simulink model "FaultOfFeeder"  (R2019a)
settings: Solver=ode1  StartTime=0.0  StopTime=2.5  FixedStep=Ts_Power  RelTol=1e-3
PostLoadFcn:
  | %% Init for wind PnO models - global system parameters
  | OVERRIDE_SSN_MEMORY_LIMIT=1;
  | Ts=50e-6;
  | % Ts=50e-10;
  | Ts_Power=Ts;
  | Ts_Control=2*Ts;
  | freq = 50;
  | Fnom=freq;
  | Vac=400e3;
InitFcn:
  | %% Init for wind PnO models - global system parameters
  | OVERRIDE_SSN_MEMORY_LIMIT=1;
  | Ts=50e-6;
  | % Ts=50e-10;
  | Ts_Power=Ts;
  | Ts_Control=2*Ts;
  | freq = 50;
  | Fnom=freq;
  | Vac=225e3;
values from neighbouring files (symbols this model uses):
  ohl_posCap = (0.01e-006)*12    (= 1.2e-07)    [variable.m]
  ohl_posInd = (1.15e-3)/12    (= 9.58333333333e-05)    [variable.m]
  ohl_posR = 0.069/12    (= 0.00575)    [variable.m]
  ohl_zeroCap = (0.004e-006)*12    (= 4.8e-08)    [variable.m]
  ohl_zeroInd = (2.86e-3)/12    (= 0.000238333333333)    [variable.m]
  ohl_zeroR = 0.1725/12    (= 0.014375)    [variable.m]
  sub_posCap = sub_posCap*6    (= 9.6e-07)    [variable.m]
  sub_posInd = sub_posInd/6    (= 0.000233333333333)    [variable.m]
  sub_posR = sub_posR/6    (= 0.006)    [variable.m]
  sub_zeroCap = sub_zeroCap*6    (= 3.84e-07)    [variable.m]
  sub_zeroInd = sub_zeroInd/6    (= 0.000583333333333)    [variable.m]
  sub_zeroR = sub_zeroR/6    (= 0.015)    [variable.m]
  transfo_L1 = 0.05999374    [variable.m]
  transfo_L2 = 0.05999374    [variable.m]
  transfo_R1 = 0.000866667    [variable.m]
  transfo_R2 = 0.00086667    [variable.m]
undefined symbols (not defined in the file or in its folder): D1, D11, Delta, den, DiscIntNeverNeededParam, dx, find_system, gcbh, num, out_Buses, out_WindFarms, sps_rtmsupport
libraries: powerlib x202, simulink x96, powerlib_meascontrol x96, elements x52, eeSinusoidalMeasurement x51, simulink_extras x42, spsVIMeasurementModel x36, eePowerMeasurement x16
(part 13 of 24)

== system FaultOfFeeder/SM_WT1/Transformer differential element 1/Differential Relay/logic block ==
  IDa1 : Inport
  IRa1 : Inport  Port=2
  IDa2 : Inport  Port=3
  IDa5 : Inport  Port=4
  Bias Characteristic - A3 : elements/Bias Characteristic  BC=[ 0 0; x1 y1; x2 y2 ]  fs=freq*32
  Data Type Conversion : DataTypeConversion  OutDataTypeStr=boolean
  Gain : Gain  Gain=c2  SaturateOnIntegerOverflow=on  OutDataTypeStr=Inherit: Same as input  ParamDataTypeStr=Inherit: Same as input
  Gain1 : Gain  Gain=c5  SaturateOnIntegerOverflow=on  OutDataTypeStr=Inherit: Same as input  ParamDataTypeStr=Inherit: Same as input
  Logical Operator : Logic  Inputs=4
  Logical Operator1 : Logic  Operator=OR
  compare{,1..3} (4 alike) : RelationalOperator  Operator=>  RndMeth=Nearest  InputSameDT=on
  pickup : Constant  Value=pickup
  unbiased : Constant  Value=unbiased
  Trip A : Outport  VectorParamsAs1DForOutWhenUnconnected=on
  wires:
  Gain/1 -> compare/1
  Gain1/1 -> compare1/1
  pickup/1 -> compare2/2
  unbiased/1 -> compare3/2
  IDa2/1 -> compare/2
  IDa5/1 -> compare1/2
  Logical Operator1/1 -> Trip A/1
  Logical Operator/1 -> Logical Operator1/1
  compare3/1 -> Logical Operator1/2
  compare/1 -> Logical Operator/2
  compare1/1 -> Logical Operator/3
  compare2/1 -> Logical Operator/4
  IRa1/1 -> Bias Characteristic - A3/2
  IDa1/1 -> Bias Characteristic - A3/1, Gain/1, Gain1/1, compare2/1, compare3/1
  Bias Characteristic - A3/1 -> Data Type Conversion/1
  Data Type Conversion/1 -> Logical Operator/1

== system FaultOfFeeder/SM_WT1/Transformer differential element 1/Differential Relay/logic block1 ==
  IDb1 : Inport
  IRb1 : Inport  Port=2
  IDb2 : Inport  Port=3
  IDb5 : Inport  Port=4
  Bias Characteristic - A3 : elements/Bias Characteristic  BC=[ 0 0; x1 y1; x2 y2 ]  fs=freq*32
  Data Type Conversion : DataTypeConversion  OutDataTypeStr=boolean
  Gain : Gain  Gain=c2  SaturateOnIntegerOverflow=on  OutDataTypeStr=Inherit: Same as input  ParamDataTypeStr=Inherit: Same as input
  Gain1 : Gain  Gain=c5  SaturateOnIntegerOverflow=on  OutDataTypeStr=Inherit: Same as input  ParamDataTypeStr=Inherit: Same as input
  Logical Operator : Logic  Inputs=4
  Logical Operator1 : Logic  Operator=OR
  compare{,1..3} (4 alike) : RelationalOperator  Operator=>  RndMeth=Nearest  InputSameDT=on
  pickup : Constant  Value=pickup
  unbiased : Constant  Value=unbiased
  Trip B : Outport  VectorParamsAs1DForOutWhenUnconnected=on
  wires:
  IDb1/1 -> compare3/1, compare2/1, Gain1/1, Gain/1, Bias Characteristic - A3/1
  IRb1/1 -> Bias Characteristic - A3/2
  compare2/1 -> Logical Operator/4
  compare1/1 -> Logical Operator/3
  compare/1 -> Logical Operator/2
  compare3/1 -> Logical Operator1/2
  Logical Operator/1 -> Logical Operator1/1
  Logical Operator1/1 -> Trip B/1
  IDb5/1 -> compare1/2
  IDb2/1 -> compare/2
  unbiased/1 -> compare3/2
  pickup/1 -> compare2/2
  Gain1/1 -> compare1/1
  Gain/1 -> compare/1
  Bias Characteristic - A3/1 -> Data Type Conversion/1
  Data Type Conversion/1 -> Logical Operator/1

== system FaultOfFeeder/SM_WT1/Transformer differential element 1/Differential Relay/logic block2 ==
  IDc1 : Inport
  IRc1 : Inport  Port=2
  IDc2 : Inport  Port=3
  IDc5 : Inport  Port=4
  Bias Characteristic - A3 : elements/Bias Characteristic  BC=[ 0 0; x1 y1; x2 y2 ]  fs=freq*32
  Data Type Conversion : DataTypeConversion  OutDataTypeStr=boolean
  Gain : Gain  Gain=c2  SaturateOnIntegerOverflow=on  OutDataTypeStr=Inherit: Same as input  ParamDataTypeStr=Inherit: Same as input
  Gain1 : Gain  Gain=c5  SaturateOnIntegerOverflow=on  OutDataTypeStr=Inherit: Same as input  ParamDataTypeStr=Inherit: Same as input
  Logical Operator : Logic  Inputs=4
  Logical Operator1 : Logic  Operator=OR
  compare{,1..3} (4 alike) : RelationalOperator  Operator=>  RndMeth=Nearest  InputSameDT=on
  pickup : Constant  Value=pickup
  unbiased : Constant  Value=unbiased
  Trip C : Outport  VectorParamsAs1DForOutWhenUnconnected=on
  wires:
  Gain/1 -> compare/1
  Gain1/1 -> compare1/1
  pickup/1 -> compare2/2
  unbiased/1 -> compare3/2
  IDc2/1 -> compare/2
  IDc5/1 -> compare1/2
  Logical Operator1/1 -> Trip C/1
  Logical Operator/1 -> Logical Operator1/1
  compare3/1 -> Logical Operator1/2
  compare/1 -> Logical Operator/2
  compare1/1 -> Logical Operator/3
  compare2/1 -> Logical Operator/4
  IRc1/1 -> Bias Characteristic - A3/2
  IDc1/1 -> Bias Characteristic - A3/1, Gain/1, Gain1/1, compare2/1, compare3/1
  Bias Characteristic - A3/1 -> Data Type Conversion/1
  Data Type Conversion/1 -> Logical Operator/1

== system FaultOfFeeder/SM_WT1/Transformer differential element 1/Signal Processing1/Differential and restraining currents ==
  IHA : Inport
  IHB : Inport  Port=2
  IHC : Inport  Port=3
  IXA : Inport  Port=4
  IXB : Inport  Port=5
  IXC : Inport  Port=6
   {,1..5} (6 alike) : elements/   fo=freq  window_size=32  harmonic=[1 2 3 4 5]
  -VG-2- : elements/-VG-2-  trtype=wye - delta  vector=1  Vh=vp  Vx=vs  nCTH=cth  nCTX=ctx
  DAB{8..12} (5 alike) : elements/DAB  filter=off  approx=Bessel  order=2  numerator=[]  denominator=[]  freq=360  resdis=off  vertres=12  xmax=10  winsize=32  G=1.0  fs=freq*32
  DAB7 : elements/DAB  filter=on  approx=Bessel  order=2  numerator=[]  denominator=[]  freq=360  resdis=off  vertres=12  xmax=10  winsize=32  G=1.0  fs=freq*32
  Terminator_{6..7,9..10,12..13,15..26} (18 alike) : Terminator
  iDa1 : Outport  VectorParamsAs1DForOutWhenUnconnected=on
  iDa2 : Outport  Port=2  VectorParamsAs1DForOutWhenUnconnected=on
  iDa5 : Outport  Port=3  VectorParamsAs1DForOutWhenUnconnected=on
  iDb1 : Outport  Port=4  VectorParamsAs1DForOutWhenUnconnected=on
  iDb2 : Outport  Port=5  VectorParamsAs1DForOutWhenUnconnected=on
  iDb5 : Outport  Port=6  VectorParamsAs1DForOutWhenUnconnected=on
  iDc1 : Outport  Port=7  VectorParamsAs1DForOutWhenUnconnected=on
  iDc2 : Outport  Port=8  VectorParamsAs1DForOutWhenUnconnected=on
  iDc5 : Outport  Port=9  VectorParamsAs1DForOutWhenUnconnected=on
  iRa1 : Outport  Port=10  VectorParamsAs1DForOutWhenUnconnected=on
  iRb1 : Outport  Port=11  VectorParamsAs1DForOutWhenUnconnected=on
  iRc1 : Outport  Port=12  VectorParamsAs1DForOutWhenUnconnected=on
  wires:
  -VG-2-/1 -> DAB7/1
  -VG-2-/2 -> DAB8/1
  -VG-2-/3 -> DAB9/1
  -VG-2-/4 -> DAB10/1
  -VG-2-/5 -> DAB11/1
  -VG-2-/6 -> DAB12/1
  " 2"/3 -> Terminator_12/1
  " 2"/4 -> Terminator_13/1
  " 4"/5 -> Terminator_21/1
  DAB9/1 -> " 2"/1
  " 5"/2 -> Terminator_26/1
  " 5"/3 -> Terminator_23/1
  " 5"/4 -> Terminator_24/1
  " 5"/5 -> Terminator_25/1
  DAB12/1 -> " 5"/1
  " 4"/3 -> Terminator_19/1
  " 4"/2 -> Terminator_22/1
  DAB11/1 -> " 4"/1
  " 4"/4 -> Terminator_20/1
  " 3"/3 -> Terminator_15/1
  " 3"/4 -> Terminator_16/1
  " 3"/5 -> Terminator_17/1
  " 3"/2 -> Terminator_18/1
  DAB10/1 -> " 3"/1
  " 2"/1 -> iDc1/1
  " 2"/2 -> iDc2/1
  " 2"/5 -> iDc5/1
  " 3"/1 -> iRa1/1
  " 4"/1 -> iRb1/1
  " 5"/1 -> iRc1/1
  IXC/1 -> -VG-2-/6
  IXB/1 -> -VG-2-/5
  IXA/1 -> -VG-2-/4
  IHC/1 -> -VG-2-/3
  IHB/1 -> -VG-2-/2
  IHA/1 -> -VG-2-/1
  " "/4 -> Terminator_6/1
  " "/3 -> Terminator_7/1
  DAB7/1 -> " "/1
  " "/1 -> iDa1/1
  " "/2 -> iDa2/1
  " "/5 -> iDa5/1
  " 1"/3 -> Terminator_9/1
  " 1"/4 -> Terminator_10/1
  " 1"/1 -> iDb1/1
  " 1"/2 -> iDb2/1
  " 1"/5 -> iDb5/1
  DAB8/1 -> " 1"/1

== system FaultOfFeeder/SM_WT1/Transformer differential element 1/Signal Processing1/Phasor-magnitude (IR) ==
  IRa1 : Inport
  IRb1 : Inport  Port=2
  IRC1 : Inport  Port=3
  Demux : Demux  Outputs=2
  Demux1 : Demux  Outputs=2
  Demux2 : Demux  Outputs=2
  Terminator_10 : Terminator
  Terminator_8 : Terminator
  Terminator_9 : Terminator
  1 freq. : Outport  VectorParamsAs1DForOutWhenUnconnected=on
  1 freq.1 : Outport  Port=2  VectorParamsAs1DForOutWhenUnconnected=on
  1 freq.2 : Outport  Port=3  VectorParamsAs1DForOutWhenUnconnected=on
  wires:
  Demux/2 -> Terminator_8/1
  Demux/1 -> 1 freq./1
  IRa1/1 -> Demux/1
  Demux1/2 -> Terminator_9/1
  Demux1/1 -> 1 freq.1/1
  IRb1/1 -> Demux1/1
  Demux2/2 -> Terminator_10/1
  Demux2/1 -> 1 freq.2/1
  IRC1/1 -> Demux2/1

== system FaultOfFeeder/SM_WT1/Transformer differential element 1/Signal Processing1/phasor-magnitude (IDa) ==
  In1 : Inport
  In2 : Inport  Port=2
  In3 : Inport  Port=3
  Demux : Demux  Outputs=2
  Demux1 : Demux  Outputs=2
  Demux2 : Demux  Outputs=2
  Terminator_11 : Terminator
  Terminator_14 : Terminator
  Terminator_8 : Terminator
  1 freq. : Outport  VectorParamsAs1DForOutWhenUnconnected=on
  2 freq. : Outport  Port=2  VectorParamsAs1DForOutWhenUnconnected=on
  5 freq. : Outport  Port=3  VectorParamsAs1DForOutWhenUnconnected=on
  wires:
  In2/1 -> Demux1/1
  In3/1 -> Demux2/1
  In1/1 -> Demux/1
  Demux1/2 -> Terminator_11/1
  Demux2/2 -> Terminator_14/1
  Demux1/1 -> 2 freq./1
  Demux2/1 -> 5 freq./1
  Demux/2 -> Terminator_8/1
  Demux/1 -> 1 freq./1

== system FaultOfFeeder/SM_WT1/Transformer differential element 1/Signal Processing1/phasor-magnitude (iDb) ==
  In1 : Inport
  In2 : Inport  Port=2
  In3 : Inport  Port=3
  Demux : Demux  Outputs=2
  Demux1 : Demux  Outputs=2
  Demux2 : Demux  Outputs=2
  Terminator_11 : Terminator
  Terminator_14 : Terminator
  Terminator_8 : Terminator
  1 freq. : Outport  VectorParamsAs1DForOutWhenUnconnected=on
  2 freq. : Outport  Port=2  VectorParamsAs1DForOutWhenUnconnected=on
  5 freq. : Outport  Port=3  VectorParamsAs1DForOutWhenUnconnected=on
  wires:
  Demux1/2 -> Terminator_11/1
  Demux2/2 -> Terminator_14/1
  Demux/2 -> Terminator_8/1
  Demux/1 -> 1 freq./1
  In1/1 -> Demux/1
  Demux1/1 -> 2 freq./1
  In2/1 -> Demux1/1
  Demux2/1 -> 5 freq./1
  In3/1 -> Demux2/1

== system FaultOfFeeder/SM_WT1/Transformer differential element 1/Signal Processing1/phasor-magnitude (iDc) ==
  In1 : Inport
  In2 : Inport  Port=2
  In3 : Inport  Port=3
  Demux : Demux  Outputs=2
  Demux1 : Demux  Outputs=2
  Demux2 : Demux  Outputs=2
  Terminator_11 : Terminator
  Terminator_14 : Terminator
  Terminator_8 : Terminator
  1 freq. : Outport  VectorParamsAs1DForOutWhenUnconnected=on
  2 freq. : Outport  Port=2  VectorParamsAs1DForOutWhenUnconnected=on
  5 freq. : Outport  Port=3  VectorParamsAs1DForOutWhenUnconnected=on
  wires:
  In3/1 -> Demux2/1
  Demux2/1 -> 5 freq./1
  In2/1 -> Demux1/1
  Demux1/1 -> 2 freq./1
  In1/1 -> Demux/1
  Demux/1 -> 1 freq./1
  Demux/2 -> Terminator_8/1
  Demux2/2 -> Terminator_14/1
  Demux1/2 -> Terminator_11/1

== system FaultOfFeeder/SM_WT1/Wind Type IV Detailed v2.1 - 1/AC fault ride though characteristic/Triggered Subsystem ==
  In1 : Inport
  Trigger : TriggerPort  VariantControl=Variant
  Time_trigger_FRT : Outport  VectorParamsAs1DForOutWhenUnconnected=on
  wires:
  In1/1 -> Time_trigger_FRT/1

== system FaultOfFeeder/SM_WT1/Wind Type IV Detailed v2.1 - 1/Control/2 sample av. ==
  in : Inport
  Delay : Delay  DelayLength=1  InitialCondition=Init_value  SampleTime=Ts
  Delay1 : Delay  DelayLength=1  InitialCondition=Init_value  SampleTime=Ts
  Gain : Gain  Gain=0.5
  Sum1 : Sum  Inputs=|++
  out : Outport
  wires:
  Gain/1 -> out/1
  in/1 -> Delay/1
  Delay1/1 -> Sum1/2
  Sum1/1 -> Gain/1
  Delay/1 -> Delay1/1, Sum1/1

== system FaultOfFeeder/SM_WT1/Wind Type IV Detailed v2.1 - 1/Control/Measurement and Transformation ==
  note: Block forever in case of
      | persistent system overvoltage
  note: Check for normal frequency
  note: Protection against unstable grid events
  note: Check for normal voltage
  note: Outputs
  note: PLL
  note: P,Q & V
  note: Inputs / filtering
  Vabc_grid : Inport
  Iabc_gc : Inport  Port=2
  IL : Inport  Port=3
  Vdc : Inport  Port=4
  Qref : Inport  Port=5
  C_var_filter : Gain  Gain=C_var_filter  SaturateOnIntegerOverflow=on  OutDataTypeStr=Inherit: Same as input  ParamDataTypeStr=Inherit: Same as input
  C_var_filter/Q : Gain  Gain=C_var_filter/Q_filter  SaturateOnIntegerOverflow=on  OutDataTypeStr=Inherit: Same as input  ParamDataTypeStr=Inherit: Same as input
  Compare To Constant1 : simulink/Logic and Bit Operations/Compare To Constant  relop=<  const=0.5  OutDataTypeStr=boolean
  Compare To Constant3 : simulink/Logic and Bit Operations/Compare To Constant  relop=<  const=0.5  OutDataTypeStr=boolean
  Constant : Constant  Value=Vnom
  Constant1 : Constant  Value=Vnom/sqrt(3)*sqrt(2)
  Constant2 : Constant  Value=20
  Constant3 : Constant  SampleTime=Ts
  Constant4 : Constant  SampleTime=Ts
  Digital Clock1 : DigitalClock  SampleTime=Ts
  Digital Clock2 : DigitalClock  SampleTime=Ts
  Discrete 3-phase PLL-Driven Positive-Sequence Active & Reactive Power : Subsystem  mask(Discrete 3-phase PLL-Driven Positive-Sequence Active & Reactive Power){Finit=freq, Fmin=freq*45/60, Par_Vinit=[Vnom/sqrt(3)*sqrt(2) 30], Par_Iinit=[Pnom/sqrt(3)/Vnom*sqrt(2) -10], Ts=Ts}
      mask prompts: Finit "Initial frequency (Hz):"; Fmin "Minimum frequency (Hz):"; Par_Vinit "Voltage initial input: [ Mag  Phase(Degrees) ]"; Par_Iinit "Current initial input: [ Mag  Phase(Degrees) ]"; Ts "Sample time:"
      mask help:
      | This discrete block measures the 3-phase active power P and reactive power Q  associated with a periodic set of 3-phase voltages and currents which may contain harmonics. P and Q are calculated by evaluating the fundamental values (positive-sequence) of the input voltages and currents with a running window over one cycle of the specified frequency (port Freq).
      |  Input port "Sin_Cos" (a two-dimension signal) provides the reference frame required for the computation.
      |
      | input 1: must give the frequency of the fundamental (Hz)
      | Input 2: must contain a  [sin(wt)  cos(wt)] two dimension signal , where w is the rotation speed (rad/s) of the reference frame used for the computation..
      | input 3: Vectorized 3-phase  instantaneous voltage (Vabc)
      | input 4: Vectorized 3-phase instantaneous current (Iabc)
      |
      | Output 1: Vector [Mag_V Mag_I] of the fundamental values (Magnitude) of the voltage & current (peak values of the positive-sequence)
      | Output 2: 3-phase PQ measurement vector [P(W) Q (var)] evaluated at the specified frequency. Current flowing into an RL circuit will produce  positive active and reactive powers.
      |
      | For the first cycle of simulation, the outputs are held constant using the values specified by the parameters "Initial input".
      | he value of the parameter "Minimum frequency" is used to determine the buffer size of the "Variable Transport Delay" block found inside this subsystem.
      mask init:
      | power_initmask();
      settings: OpenFcn=power_openblockproxy();
  Divide : Product  Inputs=*/
  Filter : Subsystem  mask{Freq=Freq_filter, Zeta=Zeta_filter, Ts=Ts}
      mask prompts: Freq "Cut-off frequency (Hz):"; Zeta "Damping factor Zeta:"; Ts "Sample time"
  Gain : Gain  Gain=1.4
  Less Than : RelationalOperator  Operator=>  OutDataTypeStr=boolean  RndMeth=Simplest
  Less Than1 : RelationalOperator  Operator=>  OutDataTypeStr=boolean  RndMeth=Simplest
  Logical Operator : Logic  AllPortsSameDT=off  OutDataTypeStr=boolean
  Math Function1 : Math  Operator=square  SaturateOnIntegerOverflow=on
  Max : MinMax  Inputs=2
  Memory : Memory  InitialCondition=1
  Second-Order Filter1 : powerlib_meascontrol/Filters/Second-Order Filter  FilterType=Lowpass  Fo=50  Zeta=0.707  Ts=Ts  Initialize=off  Vac_Init="[0,  0,  60]"  Vdc_Init=0  PlotResponse=off  FreqRange=[0, 500, 1]
      settings: SourceProductBaseCode=PS
  Selector1 : Selector  InputPortWidth=2  IndexOptions=Index vector (dialog)  Indices=1  OutputSizes=1
  Selector2 : Selector  InputPortWidth=2  IndexOptions=Index vector (dialog)  Indices=1  OutputSizes=1
  Selector3 : Selector  InputPortWidth=2  IndexOptions=Index vector (dialog)  Indices=2  OutputSizes=1
  "Sinusoidal Measurement (PLL, Three-Phase)" : eeSinusoidalMeasurement/Sinusoidal Measurement (PLL, Three-Phase)  Kp_LF=200*0.1  Ki_LF=2000*0.1  F0=freq  Theta0=0  Ts=-1
      settings: SourceProductBaseCode=PS
  Sum : Sum  Inputs=|-+
  Sum1 : Sum  Inputs=|++
  Switch1 : Switch  Criteria=u2 > Threshold
  Switch2 : Switch  Criteria=u2 > Threshold
  Terminator : Terminator
  V->pu : Gain  Gain=1/(Vnom/sqrt(3)*sqrt(2))  SaturateOnIntegerOverflow=on  OutDataTypeStr=Inherit: Same as input  ParamDataTypeStr=Inherit: Same as input
  W->pu : Gain  Gain=-1/Pnom  SaturateOnIntegerOverflow=on  OutDataTypeStr=Inherit: Same as input  ParamDataTypeStr=Inherit: Same as input
  pu->A : Gain  Gain=Pnom/sqrt(3)/Vnom*sqrt(2)  SaturateOnIntegerOverflow=on  OutDataTypeStr=Inherit: Same as input  ParamDataTypeStr=Inherit: Same as input
  pu->V : Gain  Gain=Vnom/sqrt(3)*sqrt(2)  SaturateOnIntegerOverflow=on  OutDataTypeStr=Inherit: Same as input  ParamDataTypeStr=Inherit: Same as input
  "var->pu " : Gain  Gain=-1/Pnom  SaturateOnIntegerOverflow=on  OutDataTypeStr=Inherit: Same as input  ParamDataTypeStr=Inherit: Same as input
  "IL " : Outport  VectorParamsAs1DForOutWhenUnconnected=on
  Theta_PLL : Outport  Port=2  VectorParamsAs1DForOutWhenUnconnected=on
  Pmeas : Outport  Port=3  VectorParamsAs1DForOutWhenUnconnected=on
  Qmeas : Outport  Port=4  VectorParamsAs1DForOutWhenUnconnected=on
  Vmag : Outport  Port=5  VectorParamsAs1DForOutWhenUnconnected=on
  Vdc_meas : Outport  Port=6  VectorParamsAs1DForOutWhenUnconnected=on
  Qref_pu : Outport  Port=7  VectorParamsAs1DForOutWhenUnconnected=on
  Vnormal : Outport  Port=8  VectorParamsAs1DForOutWhenUnconnected=on
  wires:
  Compare To Constant1/1 -> Switch1/2
  Switch1/1 -> Logical Operator/2  "test2"
  Less Than1/1 -> Switch1/3  "Comparator freq"
  Constant4/1 -> Switch1/1
  Digital Clock2/1 -> Compare To Constant1/1
  Switch2/1 -> Logical Operator/1  "test1"
  Less Than/1 -> Switch2/3
  Compare To Constant3/1 -> Switch2/2
  Digital Clock1/1 -> Compare To Constant3/1
  Constant3/1 -> Switch2/1
  Logical Operator/1 -> Max/1
  Max/1 -> Memory/1, [Vnormal]
  Constant/1 -> Gain/1
  Second-Order Filter1/1 -> Less Than/2
  Gain/1 -> Less Than/1
  Memory/1 -> Max/2
  [Freq] -> Less Than1/1  "Freq"
  Constant2/1 -> Less Than1/2  "20 Hz"
  [V_volt] -> Second-Order Filter1/1
  [Freq] -> Discrete 3-phase PLL-Driven Positive-Sequence Active & Reactive Power/1(Freq)
  [Vnormal] -> Vnormal/1
  [Vabc_grid] -> pu->V/1
  Selector2/1 -> [V_volt]  "V volt"
  "Sinusoidal Measurement (PLL, Three-Phase)"/3 -> Terminator/1
  [Qmeas] -> Qmeas/1
  "var->pu "/1 -> [Qmeas]  "Q meas pu"
  [PQ] -> Selector3/1
  V->pu/1 -> [Vmeas]
  [V_volt] -> V->pu/1
  Discrete 3-phase PLL-Driven Positive-Sequence Active & Reactive Power/1(Mag_V_I) -> Selector2/1
  "Sinusoidal Measurement (PLL, Three-Phase)"/1 -> [Freq]
  pu->V/1 -> Discrete 3-phase PLL-Driven Positive-Sequence Active & Reactive Power/3(Vabc)
  W->pu/1 -> [Pmeas]
  "Sinusoidal Measurement (PLL, Three-Phase)"/2 -> [Theta]
  [Theta] -> Discrete 3-phase PLL-Driven Positive-Sequence Active & Reactive Power/2(w)
  [Vabc_grid] -> "Sinusoidal Measurement (PLL, Three-Phase)"/1
  [Theta] -> Theta_PLL/1
  [Pmeas] -> Pmeas/1
  [Vmeas] -> Vmag/1
  pu->A/1 -> Discrete 3-phase PLL-Driven Positive-Sequence Active & Reactive Power/4(Iabc)
  [PQ] -> Selector1/1
  [Vdc_meas] -> Vdc_meas/1
  [Qref] -> Qref_pu/1
  [Iabc_gc] -> pu->A/1
  Discrete 3-phase PLL-Driven Positive-Sequence Active & Reactive Power/2(P_Q) -> [PQ]
  Vabc_grid/1 -> Filter/1(Vabc_grid)
  Vdc/1 -> Filter/4(Vdc)
  Qref/1 -> Filter/5(Qref)
  Filter/1("Vabc_grid ") -> [Vabc_grid]
  Filter/2("Iabc_grid_conv ") -> [Iabc_gc]
  Filter/4("Vdc ") -> [Vdc_meas]
  Filter/5("Qref ") -> [Qref]
  Iabc_gc/1 -> Filter/2(Iabc_grid_conv)
  [V_volt] -> Divide/1
  Constant1/1 -> Divide/2
  Divide/1 -> Math Function1/1
  Selector3/1 -> Sum/2  "Q grid"
  C_var_filter/1 -> Sum/1
  Sum/1 -> "var->pu "/1  "Q meas"
  Math Function1/1 -> C_var_filter/Q/1, C_var_filter/1
  Selector1/1 -> Sum1/1
  C_var_filter/Q/1 -> Sum1/2
  Sum1/1 -> W->pu/1
  IL/1 -> Filter/3(IL)
  Filter/3("IL ") -> [IL]
  [IL] -> "IL "/1

== system FaultOfFeeder/SM_WT1/Wind Type IV Detailed v2.1 - 1/Control/PI_P ==
  u : Inport
  Enable : EnablePort
  Discrete PID Controller2 : simulink/Continuous/PID Controller  Controller=PI  Form=Parallel  TimeDomain=Discrete-time  SampleTime=-1  IntegratorMethod=Forward Euler  FilterMethod=Forward Euler  ControllerParametersSource=internal  P=5  I=30  D=2  UseFilter=on  N=100  TunerSelectOption=Transfer Function Based (PID Tuner App)  InitialConditionSource=internal  InitialConditionForIntegrator=0  InitialConditionForFilter=0  DifferentiatorICPrevScaledInput=0  ExternalReset=none  TrackingMode=off  Kt=1  LimitOutput=on  UpperSaturationLimit=0.8  LowerSaturationLimit=-0.8  LinearizeAsGain=off  AntiWindupMode=none  Kb=1  POutMin=[]  POutMax=[]  IOutMin=[]  IOutMax=[]  DOutMin=[]  DOutMax=[]  NOutMin=[]  NOutMax=[]  SumOutMin=[]  SumOutMax=[]  SaturationOutMin=[]  SaturationOutMax=[]  PParamMin=[]  PParamMax=[]  IParamMin=[]  IParamMax=[]  DParamMin=[]  DParamMax=[]  NParamMin=[]  NParamMax=[]  KbParamMin=[]  KbParamMax=[]  KtParamMin=[]  KtParamMax=[]  KbOutMin=[]  KbOutMax=[]  KtOutMin=[]  KtOutMax=[]  IntegratorOutMin=[]  IntegratorOutMax=[]  FilterOutMin=[]  FilterOutMax=[]  SumI1OutMin=[]  SumI1OutMax=[]  SumI2OutMin=[]  SumI2OutMax=[]  SumI3OutMin=[]  SumI3OutMax=[]  SumI4OutMin=[]  SumI4OutMax=[]  SumDOutMin=[]  SumDOutMax=[]  DifferentiatorOutMin=[]  DifferentiatorOutMax=[]  FilterDiffOutCoefMin=[]  FilterDiffOutCoefMax=[]  ReciprocalOutMin=[]  ReciprocalOutMax=[]  SumDenOutMin=[]  SumDenOutMax=[]  SumNumOutMin=[]  SumNumOutMax=[]  DivideOutMin=[]  DivideOutMax=[]  IntegratorContinuousStateAttributes=''  IntegratorStateMustResolveToSignalObject=off  IntegratorRTWStateStorageClass=Auto  FilterContinuousStateAttributes=''  FilterStateMustResolveToSignalObject=off  FilterRTWStateStorageClass=Auto  ParallelPVariant=InternalParameters  IdealPVariant=Disabled  IVariant=InternalParameters  DVariant=Disabled  IntegratorVariant=Discrete  SatVariant=Enabled  AWVariant=Passthrough  PCopyVariant=Disabled  TRVariant=Disabled  FdbkBlocksVariant=Forward  IdealPFdbkVariant=Disabled  SatFdbkVariant=Disabled  DerivativeFilterVariant=Disabled  NVariant=Disabled  NCopyVariant=Disabled_SignalSpec  FilterICVariant=Disabled  IntegratorICVariant=InternalICs  ExternalResetVariant=Disabled  TRSumVariant=Passthrough  SumFdbkVariant=Disabled  SumVariant=Sum_PI
  PI_out : Outport  VectorParamsAs1DForOutWhenUnconnected=on
  wires:
  u/1 -> Discrete PID Controller2/1
  Discrete PID Controller2/1 -> PI_out/1  "d PI_out"

== system FaultOfFeeder/SM_WT1/Wind Type IV Detailed v2.1 - 1/Control/PI_Q ==
  Qerr : Inport
  Enable : EnablePort
  Discrete PID Controller1 : simulink/Continuous/PID Controller  Controller=PI  Form=Parallel  TimeDomain=Discrete-time  SampleTime=-1  IntegratorMethod=Forward Euler  FilterMethod=Forward Euler  ControllerParametersSource=internal  P=0.5  I=8  D=2  UseFilter=on  N=100  TunerSelectOption=Transfer Function Based (PID Tuner App)  InitialConditionSource=internal  InitialConditionForIntegrator=0  InitialConditionForFilter=0  DifferentiatorICPrevScaledInput=0  ExternalReset=none  TrackingMode=off  Kt=1  LimitOutput=off  UpperSaturationLimit=inf  LowerSaturationLimit=-inf  LinearizeAsGain=off  AntiWindupMode=none  Kb=1  POutMin=[]  POutMax=[]  IOutMin=[]  IOutMax=[]  DOutMin=[]  DOutMax=[]  NOutMin=[]  NOutMax=[]  SumOutMin=[]  SumOutMax=[]  SaturationOutMin=[]  SaturationOutMax=[]  PParamMin=[]  PParamMax=[]  IParamMin=[]  IParamMax=[]  DParamMin=[]  DParamMax=[]  NParamMin=[]  NParamMax=[]  KbParamMin=[]  KbParamMax=[]  KtParamMin=[]  KtParamMax=[]  KbOutMin=[]  KbOutMax=[]  KtOutMin=[]  KtOutMax=[]  IntegratorOutMin=[]  IntegratorOutMax=[]  FilterOutMin=[]  FilterOutMax=[]  SumI1OutMin=[]  SumI1OutMax=[]  SumI2OutMin=[]  SumI2OutMax=[]  SumI3OutMin=[]  SumI3OutMax=[]  SumI4OutMin=[]  SumI4OutMax=[]  SumDOutMin=[]  SumDOutMax=[]  DifferentiatorOutMin=[]  DifferentiatorOutMax=[]  FilterDiffOutCoefMin=[]  FilterDiffOutCoefMax=[]  ReciprocalOutMin=[]  ReciprocalOutMax=[]  SumDenOutMin=[]  SumDenOutMax=[]  SumNumOutMin=[]  SumNumOutMax=[]  DivideOutMin=[]  DivideOutMax=[]  IntegratorContinuousStateAttributes=''  IntegratorStateMustResolveToSignalObject=off  IntegratorRTWStateStorageClass=Auto  FilterContinuousStateAttributes=''  FilterStateMustResolveToSignalObject=off  FilterRTWStateStorageClass=Auto  ParallelPVariant=InternalParameters  IdealPVariant=Disabled  IVariant=InternalParameters  DVariant=Disabled  IntegratorVariant=Discrete  SatVariant=Disabled  AWVariant=Passthrough  PCopyVariant=Disabled  TRVariant=Disabled  FdbkBlocksVariant=Forward  IdealPFdbkVariant=Disabled  SatFdbkVariant=Disabled  DerivativeFilterVariant=Disabled  NVariant=Disabled  NCopyVariant=Disabled_SignalSpec  FilterICVariant=Disabled  IntegratorICVariant=InternalICs  ExternalResetVariant=Disabled  TRSumVariant=Passthrough  SumFdbkVariant=Disabled  SumVariant=Sum_PI
  PI_out : Outport  VectorParamsAs1DForOutWhenUnconnected=on
  wires:
  Qerr/1 -> Discrete PID Controller1/1
  Discrete PID Controller1/1 -> PI_out/1  "q PI_out"

== system FaultOfFeeder/SM_WT1/Wind Type IV Detailed v2.1 - 1/Control/Pulse Generator1 ==
  Duty_Cycle : Inport
  Add : Sum  Inputs=-+
  Constant3 : Constant
  Constant4 : Constant  Value=0
  Digital Clock : DigitalClock  SampleTime=Ts
  Divide2 : Product  Inputs=**
  Divide3 : Product  Inputs=**
  Math Function : Math  Operator=mod  SaturateOnIntegerOverflow=on
  Nb_of_samples_by_cycle : Constant  Value=1/Freq_sawtooth/Ts
  Relational Operator1 : RelationalOperator  Operator=>  OutDataTypeStr=boolean  RndMeth=Nearest
  Rounding Function1 : Rounding  Operator=round
  Switch : Switch  Threshold=0.5
  Ts : Constant  Value=Ts
  Pulse : Outport  VectorParamsAs1DForOutWhenUnconnected=on
  wires:
  Math Function/1 -> Relational Operator1/2
  Constant4/1 -> Switch/3
  Constant3/1 -> Switch/1
  Relational Operator1/1 -> Switch/2
  Nb_of_samples_by_cycle/1 -> Rounding Function1/1
  Divide2/1 -> Relational Operator1/1
  Divide3/1 -> Add/2, Math Function/2  "Period_of_cycle"
  Duty_Cycle/1 -> Divide2/1
  Rounding Function1/1 -> Divide3/2  "Nb_of_samples_by_cycle"
  Ts/1 -> Divide3/1, Add/1
  Digital Clock/1 -> Math Function/1
  Add/1 -> Divide2/2
  Switch/1 -> Pulse/1

== system FaultOfFeeder/SM_WT1/Wind Type IV Detailed v2.1 - 2/AC fault ride though characteristic/Triggered Subsystem ==
  In1 : Inport
  Trigger : TriggerPort  VariantControl=Variant
  Time_trigger_FRT : Outport  VectorParamsAs1DForOutWhenUnconnected=on
  wires:
  In1/1 -> Time_trigger_FRT/1

== system FaultOfFeeder/SM_WT1/Wind Type IV Detailed v2.1 - 2/Control/2 sample av. ==
  in : Inport
  Delay : Delay  DelayLength=1  InitialCondition=Init_value  SampleTime=Ts
  Delay1 : Delay  DelayLength=1  InitialCondition=Init_value  SampleTime=Ts
  Gain : Gain  Gain=0.5
  Sum1 : Sum  Inputs=|++
  out : Outport
  wires:
  Delay/1 -> Sum1/1, Delay1/1
  Sum1/1 -> Gain/1
  Delay1/1 -> Sum1/2
  in/1 -> Delay/1
  Gain/1 -> out/1

== system FaultOfFeeder/SM_WT1/Wind Type IV Detailed v2.1 - 2/Control/Measurement and Transformation ==
  note: Inputs / filtering
  note: P,Q & V
  note: PLL
  note: Outputs
  note: Check for normal voltage
  note: Protection against unstable grid events
  note: Check for normal frequency
  note: Block forever in case of
      | persistent system overvoltage
  Vabc_grid : Inport
  Iabc_gc : Inport  Port=2
  IL : Inport  Port=3
  Vdc : Inport  Port=4
  Qref : Inport  Port=5
  C_var_filter : Gain  Gain=C_var_filter  SaturateOnIntegerOverflow=on  OutDataTypeStr=Inherit: Same as input  ParamDataTypeStr=Inherit: Same as input
  C_var_filter/Q : Gain  Gain=C_var_filter/Q_filter  SaturateOnIntegerOverflow=on  OutDataTypeStr=Inherit: Same as input  ParamDataTypeStr=Inherit: Same as input
  Compare To Constant1 : simulink/Logic and Bit Operations/Compare To Constant  relop=<  const=0.5  OutDataTypeStr=boolean
  Compare To Constant3 : simulink/Logic and Bit Operations/Compare To Constant  relop=<  const=0.5  OutDataTypeStr=boolean
  Constant : Constant  Value=Vnom
  Constant1 : Constant  Value=Vnom/sqrt(3)*sqrt(2)
  Constant2 : Constant  Value=20
  Constant3 : Constant  SampleTime=Ts
  Constant4 : Constant  SampleTime=Ts
  Digital Clock1 : DigitalClock  SampleTime=Ts
  Digital Clock2 : DigitalClock  SampleTime=Ts
  Discrete 3-phase PLL-Driven Positive-Sequence Active & Reactive Power : Subsystem  mask(Discrete 3-phase PLL-Driven Positive-Sequence Active & Reactive Power){Finit=freq, Fmin=freq*45/60, Par_Vinit=[Vnom/sqrt(3)*sqrt(2) 30], Par_Iinit=[Pnom/sqrt(3)/Vnom*sqrt(2) -10], Ts=Ts}
      mask prompts: Finit "Initial frequency (Hz):"; Fmin "Minimum frequency (Hz):"; Par_Vinit "Voltage initial input: [ Mag  Phase(Degrees) ]"; Par_Iinit "Current initial input: [ Mag  Phase(Degrees) ]"; Ts "Sample time:"
      mask help:
      | This discrete block measures the 3-phase active power P and reactive power Q  associated with a periodic set of 3-phase voltages and currents which may contain harmonics. P and Q are calculated by evaluating the fundamental values (positive-sequence) of the input voltages and currents with a running window over one cycle of the specified frequency (port Freq).
      |  Input port "Sin_Cos" (a two-dimension signal) provides the reference frame required for the computation.
      |
      | input 1: must give the frequency of the fundamental (Hz)
      | Input 2: must contain a  [sin(wt)  cos(wt)] two dimension signal , where w is the rotation speed (rad/s) of the reference frame used for the computation..
      | input 3: Vectorized 3-phase  instantaneous voltage (Vabc)
      | input 4: Vectorized 3-phase instantaneous current (Iabc)
      |
      | Output 1: Vector [Mag_V Mag_I] of the fundamental values (Magnitude) of the voltage & current (peak values of the positive-sequence)
      | Output 2: 3-phase PQ measurement vector [P(W) Q (var)] evaluated at the specified frequency. Current flowing into an RL circuit will produce  positive active and reactive powers.
      |
      | For the first cycle of simulation, the outputs are held constant using the values specified by the parameters "Initial input".
      | he value of the parameter "Minimum frequency" is used to determine the buffer size of the "Variable Transport Delay" block found inside this subsystem.
      mask init:
      | power_initmask();
      settings: OpenFcn=power_openblockproxy();
  Divide : Product  Inputs=*/
  Filter : Subsystem  mask{Freq=Freq_filter, Zeta=Zeta_filter, Ts=Ts}
      mask prompts: Freq "Cut-off frequency (Hz):"; Zeta "Damping factor Zeta:"; Ts "Sample time"
  Gain : Gain  Gain=1.4
  Less Than : RelationalOperator  Operator=>  OutDataTypeStr=boolean  RndMeth=Simplest
  Less Than1 : RelationalOperator  Operator=>  OutDataTypeStr=boolean  RndMeth=Simplest
  Logical Operator : Logic  AllPortsSameDT=off  OutDataTypeStr=boolean
  Math Function1 : Math  Operator=square  SaturateOnIntegerOverflow=on
  Max : MinMax  Inputs=2
  Memory : Memory  InitialCondition=1
  Second-Order Filter1 : powerlib_meascontrol/Filters/Second-Order Filter  FilterType=Lowpass  Fo=50  Zeta=0.707  Ts=Ts  Initialize=off  Vac_Init="[0,  0,  60]"  Vdc_Init=0  PlotResponse=off  FreqRange=[0, 500, 1]
      settings: SourceProductBaseCode=PS
  Selector1 : Selector  InputPortWidth=2  IndexOptions=Index vector (dialog)  Indices=1  OutputSizes=1
  Selector2 : Selector  InputPortWidth=2  IndexOptions=Index vector (dialog)  Indices=1  OutputSizes=1
  Selector3 : Selector  InputPortWidth=2  IndexOptions=Index vector (dialog)  Indices=2  OutputSizes=1
  "Sinusoidal Measurement (PLL, Three-Phase)" : eeSinusoidalMeasurement/Sinusoidal Measurement (PLL, Three-Phase)  Kp_LF=200*0.1  Ki_LF=2000*0.1  F0=freq  Theta0=0  Ts=-1
      settings: SourceProductBaseCode=PS
  Sum : Sum  Inputs=|-+
  Sum1 : Sum  Inputs=|++
  Switch1 : Switch  Criteria=u2 > Threshold
  Switch2 : Switch  Criteria=u2 > Threshold
  Terminator : Terminator
  V->pu : Gain  Gain=1/(Vnom/sqrt(3)*sqrt(2))  SaturateOnIntegerOverflow=on  OutDataTypeStr=Inherit: Same as input  ParamDataTypeStr=Inherit: Same as input
  W->pu : Gain  Gain=-1/Pnom  SaturateOnIntegerOverflow=on  OutDataTypeStr=Inherit: Same as input  ParamDataTypeStr=Inherit: Same as input
  pu->A : Gain  Gain=Pnom/sqrt(3)/Vnom*sqrt(2)  SaturateOnIntegerOverflow=on  OutDataTypeStr=Inherit: Same as input  ParamDataTypeStr=Inherit: Same as input
  pu->V : Gain  Gain=Vnom/sqrt(3)*sqrt(2)  SaturateOnIntegerOverflow=on  OutDataTypeStr=Inherit: Same as input  ParamDataTypeStr=Inherit: Same as input
  "var->pu " : Gain  Gain=-1/Pnom  SaturateOnIntegerOverflow=on  OutDataTypeStr=Inherit: Same as input  ParamDataTypeStr=Inherit: Same as input
  "IL " : Outport  VectorParamsAs1DForOutWhenUnconnected=on
  Theta_PLL : Outport  Port=2  VectorParamsAs1DForOutWhenUnconnected=on
  Pmeas : Outport  Port=3  VectorParamsAs1DForOutWhenUnconnected=on
  Qmeas : Outport  Port=4  VectorParamsAs1DForOutWhenUnconnected=on
  Vmag : Outport  Port=5  VectorParamsAs1DForOutWhenUnconnected=on
  Vdc_meas : Outport  Port=6  VectorParamsAs1DForOutWhenUnconnected=on
  Qref_pu : Outport  Port=7  VectorParamsAs1DForOutWhenUnconnected=on
  Vnormal : Outport  Port=8  VectorParamsAs1DForOutWhenUnconnected=on
  wires:
  [IL] -> "IL "/1
  Filter/3("IL ") -> [IL]
  IL/1 -> Filter/3(IL)
  Sum1/1 -> W->pu/1
  C_var_filter/Q/1 -> Sum1/2
  Selector1/1 -> Sum1/1
  Math Function1/1 -> C_var_filter/1, C_var_filter/Q/1
  Sum/1 -> "var->pu "/1  "Q meas"
  C_var_filter/1 -> Sum/1
  Selector3/1 -> Sum/2  "Q grid"
  Divide/1 -> Math Function1/1
  Constant1/1 -> Divide/2
  [V_volt] -> Divide/1
  Iabc_gc/1 -> Filter/2(Iabc_grid_conv)
  Filter/5("Qref ") -> [Qref]
  Filter/4("Vdc ") -> [Vdc_meas]
  Filter/2("Iabc_grid_conv ") -> [Iabc_gc]
  Filter/1("Vabc_grid ") -> [Vabc_grid]
  Qref/1 -> Filter/5(Qref)
  Vdc/1 -> Filter/4(Vdc)
  Vabc_grid/1 -> Filter/1(Vabc_grid)
  Discrete 3-phase PLL-Driven Positive-Sequence Active & Reactive Power/2(P_Q) -> [PQ]
  [Iabc_gc] -> pu->A/1
  [Qref] -> Qref_pu/1
  [Vdc_meas] -> Vdc_meas/1
  [PQ] -> Selector1/1
  pu->A/1 -> Discrete 3-phase PLL-Driven Positive-Sequence Active & Reactive Power/4(Iabc)
  [Vmeas] -> Vmag/1
  [Pmeas] -> Pmeas/1
  [Theta] -> Theta_PLL/1
  [Vabc_grid] -> "Sinusoidal Measurement (PLL, Three-Phase)"/1
  [Theta] -> Discrete 3-phase PLL-Driven Positive-Sequence Active & Reactive Power/2(w)
  "Sinusoidal Measurement (PLL, Three-Phase)"/2 -> [Theta]
  W->pu/1 -> [Pmeas]
  pu->V/1 -> Discrete 3-phase PLL-Driven Positive-Sequence Active & Reactive Power/3(Vabc)
  "Sinusoidal Measurement (PLL, Three-Phase)"/1 -> [Freq]
  Discrete 3-phase PLL-Driven Positive-Sequence Active & Reactive Power/1(Mag_V_I) -> Selector2/1
  [V_volt] -> V->pu/1
  V->pu/1 -> [Vmeas]
  [PQ] -> Selector3/1
  "var->pu "/1 -> [Qmeas]  "Q meas pu"
  [Qmeas] -> Qmeas/1
  "Sinusoidal Measurement (PLL, Three-Phase)"/3 -> Terminator/1
  Selector2/1 -> [V_volt]  "V volt"
  [Vabc_grid] -> pu->V/1
  [Vnormal] -> Vnormal/1
  [Freq] -> Discrete 3-phase PLL-Driven Positive-Sequence Active & Reactive Power/1(Freq)
  [V_volt] -> Second-Order Filter1/1
  Constant2/1 -> Less Than1/2  "20 Hz"
  [Freq] -> Less Than1/1  "Freq"
  Memory/1 -> Max/2
  Gain/1 -> Less Than/1
  Second-Order Filter1/1 -> Less Than/2
  Constant/1 -> Gain/1
  Max/1 -> [Vnormal], Memory/1
  Logical Operator/1 -> Max/1
  Constant3/1 -> Switch2/1
  Digital Clock1/1 -> Compare To Constant3/1
  Compare To Constant3/1 -> Switch2/2
  Less Than/1 -> Switch2/3
  Switch2/1 -> Logical Operator/1  "test1"
  Digital Clock2/1 -> Compare To Constant1/1
  Constant4/1 -> Switch1/1
  Less Than1/1 -> Switch1/3  "Comparator freq"
  Switch1/1 -> Logical Operator/2  "test2"
  Compare To Constant1/1 -> Switch1/2

== system FaultOfFeeder/SM_WT1/Wind Type IV Detailed v2.1 - 2/Control/PI_P ==
  u : Inport
  Enable : EnablePort
  Discrete PID Controller2 : simulink/Continuous/PID Controller  Controller=PI  Form=Parallel  TimeDomain=Discrete-time  SampleTime=-1  IntegratorMethod=Forward Euler  FilterMethod=Forward Euler  ControllerParametersSource=internal  P=5  I=30  D=2  UseFilter=on  N=100  TunerSelectOption=Transfer Function Based (PID Tuner App)  InitialConditionSource=internal  InitialConditionForIntegrator=0  InitialConditionForFilter=0  DifferentiatorICPrevScaledInput=0  ExternalReset=none  TrackingMode=off  Kt=1  LimitOutput=on  UpperSaturationLimit=0.8  LowerSaturationLimit=-0.8  LinearizeAsGain=off  AntiWindupMode=none  Kb=1  POutMin=[]  POutMax=[]  IOutMin=[]  IOutMax=[]  DOutMin=[]  DOutMax=[]  NOutMin=[]  NOutMax=[]  SumOutMin=[]  SumOutMax=[]  SaturationOutMin=[]  SaturationOutMax=[]  PParamMin=[]  PParamMax=[]  IParamMin=[]  IParamMax=[]  DParamMin=[]  DParamMax=[]  NParamMin=[]  NParamMax=[]  KbParamMin=[]  KbParamMax=[]  KtParamMin=[]  KtParamMax=[]  KbOutMin=[]  KbOutMax=[]  KtOutMin=[]  KtOutMax=[]  IntegratorOutMin=[]  IntegratorOutMax=[]  FilterOutMin=[]  FilterOutMax=[]  SumI1OutMin=[]  SumI1OutMax=[]  SumI2OutMin=[]  SumI2OutMax=[]  SumI3OutMin=[]  SumI3OutMax=[]  SumI4OutMin=[]  SumI4OutMax=[]  SumDOutMin=[]  SumDOutMax=[]  DifferentiatorOutMin=[]  DifferentiatorOutMax=[]  FilterDiffOutCoefMin=[]  FilterDiffOutCoefMax=[]  ReciprocalOutMin=[]  ReciprocalOutMax=[]  SumDenOutMin=[]  SumDenOutMax=[]  SumNumOutMin=[]  SumNumOutMax=[]  DivideOutMin=[]  DivideOutMax=[]  IntegratorContinuousStateAttributes=''  IntegratorStateMustResolveToSignalObject=off  IntegratorRTWStateStorageClass=Auto  FilterContinuousStateAttributes=''  FilterStateMustResolveToSignalObject=off  FilterRTWStateStorageClass=Auto  ParallelPVariant=InternalParameters  IdealPVariant=Disabled  IVariant=InternalParameters  DVariant=Disabled  IntegratorVariant=Discrete  SatVariant=Enabled  AWVariant=Passthrough  PCopyVariant=Disabled  TRVariant=Disabled  FdbkBlocksVariant=Forward  IdealPFdbkVariant=Disabled  SatFdbkVariant=Disabled  DerivativeFilterVariant=Disabled  NVariant=Disabled  NCopyVariant=Disabled_SignalSpec  FilterICVariant=Disabled  IntegratorICVariant=InternalICs  ExternalResetVariant=Disabled  TRSumVariant=Passthrough  SumFdbkVariant=Disabled  SumVariant=Sum_PI
  PI_out : Outport  VectorParamsAs1DForOutWhenUnconnected=on
  wires:
  Discrete PID Controller2/1 -> PI_out/1  "d PI_out"
  u/1 -> Discrete PID Controller2/1

== system FaultOfFeeder/SM_WT1/Wind Type IV Detailed v2.1 - 2/Control/PI_Q ==
  Qerr : Inport
  Enable : EnablePort
  Discrete PID Controller1 : simulink/Continuous/PID Controller  Controller=PI  Form=Parallel  TimeDomain=Discrete-time  SampleTime=-1  IntegratorMethod=Forward Euler  FilterMethod=Forward Euler  ControllerParametersSource=internal  P=0.5  I=8  D=2  UseFilter=on  N=100  TunerSelectOption=Transfer Function Based (PID Tuner App)  InitialConditionSource=internal  InitialConditionForIntegrator=0  InitialConditionForFilter=0  DifferentiatorICPrevScaledInput=0  ExternalReset=none  TrackingMode=off  Kt=1  LimitOutput=off  UpperSaturationLimit=inf  LowerSaturationLimit=-inf  LinearizeAsGain=off  AntiWindupMode=none  Kb=1  POutMin=[]  POutMax=[]  IOutMin=[]  IOutMax=[]  DOutMin=[]  DOutMax=[]  NOutMin=[]  NOutMax=[]  SumOutMin=[]  SumOutMax=[]  SaturationOutMin=[]  SaturationOutMax=[]  PParamMin=[]  PParamMax=[]  IParamMin=[]  IParamMax=[]  DParamMin=[]  DParamMax=[]  NParamMin=[]  NParamMax=[]  KbParamMin=[]  KbParamMax=[]  KtParamMin=[]  KtParamMax=[]  KbOutMin=[]  KbOutMax=[]  KtOutMin=[]  KtOutMax=[]  IntegratorOutMin=[]  IntegratorOutMax=[]  FilterOutMin=[]  FilterOutMax=[]  SumI1OutMin=[]  SumI1OutMax=[]  SumI2OutMin=[]  SumI2OutMax=[]  SumI3OutMin=[]  SumI3OutMax=[]  SumI4OutMin=[]  SumI4OutMax=[]  SumDOutMin=[]  SumDOutMax=[]  DifferentiatorOutMin=[]  DifferentiatorOutMax=[]  FilterDiffOutCoefMin=[]  FilterDiffOutCoefMax=[]  ReciprocalOutMin=[]  ReciprocalOutMax=[]  SumDenOutMin=[]  SumDenOutMax=[]  SumNumOutMin=[]  SumNumOutMax=[]  DivideOutMin=[]  DivideOutMax=[]  IntegratorContinuousStateAttributes=''  IntegratorStateMustResolveToSignalObject=off  IntegratorRTWStateStorageClass=Auto  FilterContinuousStateAttributes=''  FilterStateMustResolveToSignalObject=off  FilterRTWStateStorageClass=Auto  ParallelPVariant=InternalParameters  IdealPVariant=Disabled  IVariant=InternalParameters  DVariant=Disabled  IntegratorVariant=Discrete  SatVariant=Disabled  AWVariant=Passthrough  PCopyVariant=Disabled  TRVariant=Disabled  FdbkBlocksVariant=Forward  IdealPFdbkVariant=Disabled  SatFdbkVariant=Disabled  DerivativeFilterVariant=Disabled  NVariant=Disabled  NCopyVariant=Disabled_SignalSpec  FilterICVariant=Disabled  IntegratorICVariant=InternalICs  ExternalResetVariant=Disabled  TRSumVariant=Passthrough  SumFdbkVariant=Disabled  SumVariant=Sum_PI
  PI_out : Outport  VectorParamsAs1DForOutWhenUnconnected=on
  wires:
  Discrete PID Controller1/1 -> PI_out/1  "q PI_out"
  Qerr/1 -> Discrete PID Controller1/1

== system FaultOfFeeder/SM_WT1/Wind Type IV Detailed v2.1 - 2/Control/Pulse Generator1 ==
  Duty_Cycle : Inport
  Add : Sum  Inputs=-+
  Constant3 : Constant
  Constant4 : Constant  Value=0
  Digital Clock : DigitalClock  SampleTime=Ts
  Divide2 : Product  Inputs=**
  Divide3 : Product  Inputs=**
  Math Function : Math  Operator=mod  SaturateOnIntegerOverflow=on
  Nb_of_samples_by_cycle : Constant  Value=1/Freq_sawtooth/Ts
  Relational Operator1 : RelationalOperator  Operator=>  OutDataTypeStr=boolean  RndMeth=Nearest
  Rounding Function1 : Rounding  Operator=round
  Switch : Switch  Threshold=0.5
  Ts : Constant  Value=Ts
  Pulse : Outport  VectorParamsAs1DForOutWhenUnconnected=on
  wires:
  Switch/1 -> Pulse/1
  Add/1 -> Divide2/2
  Digital Clock/1 -> Math Function/1
  Ts/1 -> Add/1, Divide3/1
  Rounding Function1/1 -> Divide3/2  "Nb_of_samples_by_cycle"
  Duty_Cycle/1 -> Divide2/1
  Divide3/1 -> Math Function/2, Add/2  "Period_of_cycle"
  Divide2/1 -> Relational Operator1/1
  Nb_of_samples_by_cycle/1 -> Rounding Function1/1
  Relational Operator1/1 -> Switch/2
  Constant3/1 -> Switch/1
  Constant4/1 -> Switch/3
  Math Function/1 -> Relational Operator1/2

== system FaultOfFeeder/SM_WT1/Wind Type IV Detailed v2.1 - 3/AC fault ride though characteristic/Triggered Subsystem ==
  In1 : Inport
  Trigger : TriggerPort  VariantControl=Variant
  Time_trigger_FRT : Outport  VectorParamsAs1DForOutWhenUnconnected=on
  wires:
  In1/1 -> Time_trigger_FRT/1

== system FaultOfFeeder/SM_WT1/Wind Type IV Detailed v2.1 - 3/Control/2 sample av. ==
  in : Inport
  Delay : Delay  DelayLength=1  InitialCondition=Init_value  SampleTime=Ts
  Delay1 : Delay  DelayLength=1  InitialCondition=Init_value  SampleTime=Ts
  Gain : Gain  Gain=0.5
  Sum1 : Sum  Inputs=|++
  out : Outport
  wires:
  Delay/1 -> Sum1/1, Delay1/1
  Sum1/1 -> Gain/1
  Delay1/1 -> Sum1/2
  in/1 -> Delay/1
  Gain/1 -> out/1
